simulink model "foot_trajectory"  (R2021a)
settings: Solver=ode15s  StartTime=0.0  StopTime=20  EnableMultiTasking=on
undefined symbols (not defined in the file): C, com_initial_height, H, Kvec, L, L1, L2, L3, leg1, leg2, leg3, leg4, q0, q0_leg1, q0_leg2, q0_leg3, q0_leg4, X, Y, Z
libraries: sm_lib x52, nesl_utility x28, roblocks x8, simulink_extras x1
(part 3 of 3)

== matlab function foot_trajectory/pInv/getJinv ==
  data: J1 input; Jinv output; J2 input; J3 input; J4 input
function Jinv = getJinv(J1, J2, J3, J4)

% Preciso revisar essa parte, e como montar o jacobiano.
% definir se uso parametro 'trans' ou 'rot' do jacbo0() pra extrair as partes que eu quiser

% --- Monta jacobiano blocado diag{J1,J2,J3,J4} (12x12) ------------------
J = blkdiag(J1,J2,J3,J4);

% posso testar inv(J) se quadrada
% posso testar pinv(J)
Jinv = inv(J);
